simulink model "xy_platforma_fuzzy_test"  (Simulink 7.5)
settings: Solver=ode45  StartTime=0.0  StopTime=t_sim  RelTol=1e-3
values from neighbouring files (symbols this model uses):
  g = 9.81    [helikopter_maketa_paraametri.m]    (also in helikopter_maketa_parametri.m)
  Td = 0.1    [proo.m]
undefined symbols (not defined in the file or in its folder): a, ak_x, ak_y, Ax, Ay, const, d, Fc, freq_x, freq_y, Fs, Jl, K, K_komp, l, ml, period_x, period_y, phase_x, phase_y, phasedelay_x, phasedelay_y, pw_x, pw_y, R, r, t_step, vs, x0, x_poc_poz, x_step, y0, y_poc_poz, y_step
libraries: simulink x18, fuzblock x2
settings Model: Creator=Damjan  LastModifiedBy=Miha
settings DebuggingCC: SolverPrmCheckMsg=none

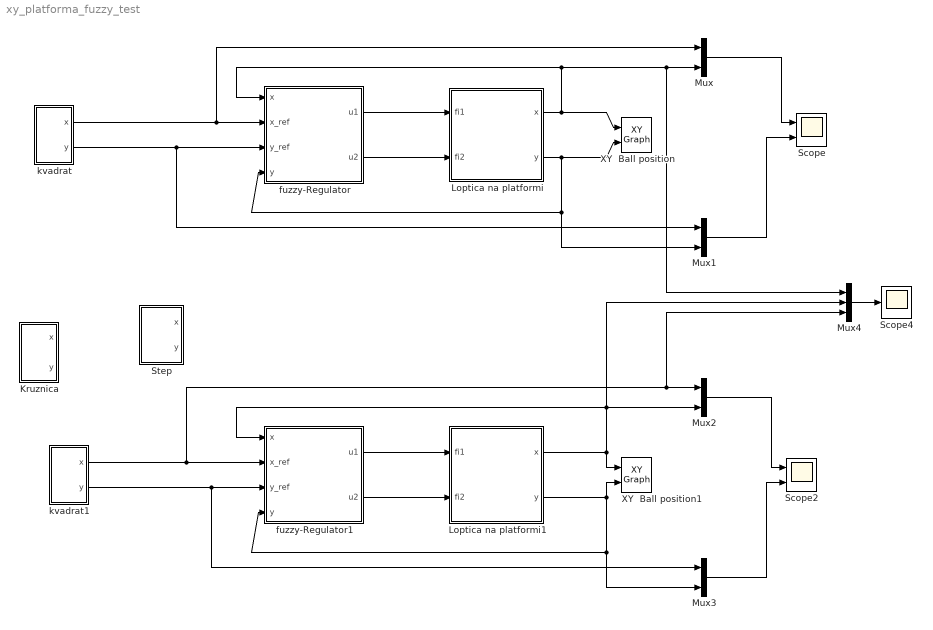
== system xy_platforma_fuzzy_test ==
  Kruznica : Subsystem
  Loptica na platformi : Subsystem
  Loptica na platformi1 : Subsystem
  Mux{,1..3} (4 alike) : Mux  Inputs=2
  Mux4 : Mux  Inputs=3
  Scope : Scope  NumInputPorts=2
      settings: YMin=0.15~0.15  YMax=0.2025~0.2025  SampleInput=on  SampleTime=1/25
  Scope2 : Scope  NumInputPorts=2
      settings: YMin=0.06~0.07  YMax=0.2~0.2  SaveName=ScopeData2  SampleInput=on  SampleTime=1/25
  Scope4 : Scope
      settings: TimeRange=4.054054054054055  YMin=0.115  YMax=0.22  SaveName=step  DataFormat=Array  MaxDataPoints=50000
  Step : Subsystem
  XY  Ball position : simulink/Sinks/XY Graph  SystemSampleTime=-1  xmin=0  xmax=0.3  ymin=0  ymax=0.3  st=-1
  XY  Ball position1 : simulink/Sinks/XY Graph  SystemSampleTime=-1  xmin=0  xmax=0.3  ymin=0  ymax=0.3  st=-1
  fuzzy-Regulator : Subsystem
  fuzzy-Regulator1 : Subsystem
  kvadrat : Subsystem
  kvadrat1 : Subsystem
  wires:
  Loptica na platformi/1(x) -> XY  Ball position/1, fuzzy-Regulator/1(x), Mux/2, Mux4/1
  Loptica na platformi/2(y) -> XY  Ball position/2, fuzzy-Regulator/4(y), Mux1/2
  Mux/1 -> Scope/1
  Mux1/1 -> Scope/2
  fuzzy-Regulator/1(u1) -> Loptica na platformi/1(fi1)
  fuzzy-Regulator/2(u2) -> Loptica na platformi/2(fi2)
  Loptica na platformi1/1(x) -> XY  Ball position1/1, fuzzy-Regulator1/1(x), Mux2/2, Mux4/2
  Loptica na platformi1/2(y) -> XY  Ball position1/2, fuzzy-Regulator1/4(y), Mux3/2
  Mux2/1 -> Scope2/1
  Mux3/1 -> Scope2/2
  fuzzy-Regulator1/1(u1) -> Loptica na platformi1/1(fi1)
  fuzzy-Regulator1/2(u2) -> Loptica na platformi1/2(fi2)
  kvadrat1/1(x) -> fuzzy-Regulator1/2(x_ref), Mux2/1, Mux4/3
  kvadrat1/2(y) -> fuzzy-Regulator1/3(y_ref), Mux3/1
  Mux4/1 -> Scope4/1
  kvadrat/1(x) -> fuzzy-Regulator/2(x_ref), Mux/1
  kvadrat/2(y) -> fuzzy-Regulator/3(y_ref), Mux1/1

== system xy_platforma_fuzzy_test/Kruznica ==
  sin x2 : Sin  Amplitude=Ax  Bias=x0  Frequency=freq_x  Phase=phase_x  Samples=10  SampleTime=0  Offset=0
  sin y2 : Sin  Amplitude=Ay  Bias=y0  Frequency=freq_y  Phase=phase_y  Samples=10  SampleTime=0  Offset=0
  x : Outport
  y : Outport  Port=2
  wires:
  sin x2/1 -> x/1
  sin y2/1 -> y/1

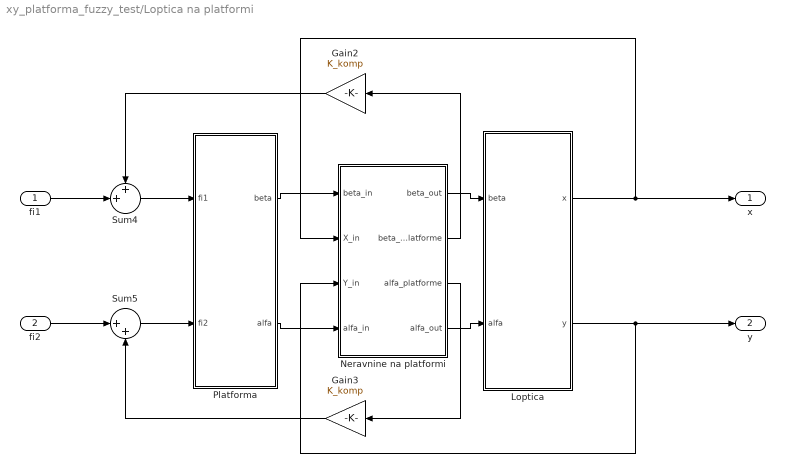
== system xy_platforma_fuzzy_test/Loptica na platformi ==
  fi1 : Inport
  fi2 : Inport  Port=2
  Gain2 : Gain  Gain=K_komp
  Gain3 : Gain  Gain=K_komp
  Loptica : Subsystem
  Neravnine na platformi : Subsystem
  Platforma : Subsystem
  Sum4 : Sum  Inputs=++|  RndMeth=Nearest
  Sum5 : Sum  Inputs=|++  RndMeth=Nearest
  x : Outport
  y : Outport  Port=2
  wires:
  Loptica/1(x) -> x/1, Neravnine na platformi/2(X_in)
  Platforma/1(beta) -> Neravnine na platformi/1(" beta_in")
  Platforma/2(alfa) -> Neravnine na platformi/4(alfa_in)
  Sum4/1 -> Platforma/1(fi1)
  Sum5/1 -> Platforma/2(fi2)
  Neravnine na platformi/3(alfa_platforme) -> Gain3/1
  Neravnine na platformi/2(beta_platforme) -> Gain2/1
  Loptica/2(y) -> y/1, Neravnine na platformi/3(Y_in)
  Neravnine na platformi/4(alfa_out) -> Loptica/2(alfa)
  Neravnine na platformi/1(beta_out) -> Loptica/1(beta)
  fi1/1 -> Sum4/2
  fi2/1 -> Sum5/1
  Gain2/1 -> Sum4/1
  Gain3/1 -> Sum5/2

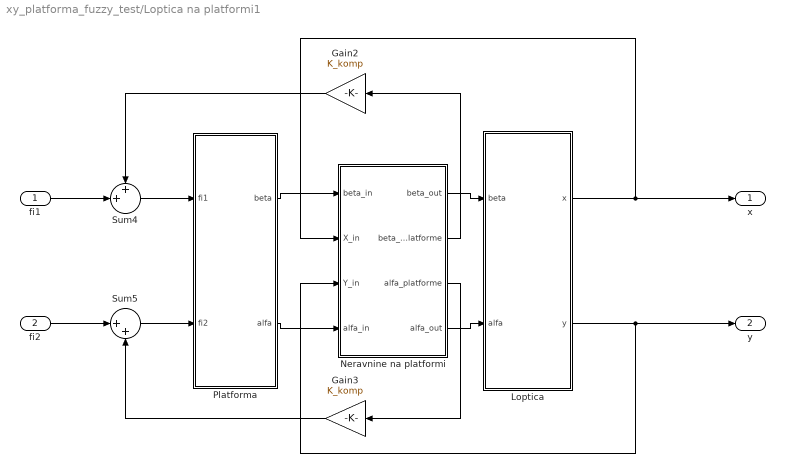
== system xy_platforma_fuzzy_test/Loptica na platformi1 ==
  fi1 : Inport
  fi2 : Inport  Port=2
  Gain2 : Gain  Gain=K_komp
  Gain3 : Gain  Gain=K_komp
  Loptica : Subsystem
  Neravnine na platformi : Subsystem
  Platforma : Subsystem
  Sum4 : Sum  Inputs=++|  RndMeth=Nearest
  Sum5 : Sum  Inputs=|++  RndMeth=Nearest
  x : Outport
  y : Outport  Port=2
  wires:
  Loptica/1(x) -> x/1, Neravnine na platformi/2(X_in)
  Platforma/1(beta) -> Neravnine na platformi/1(" beta_in")
  Platforma/2(alfa) -> Neravnine na platformi/4(alfa_in)
  Sum4/1 -> Platforma/1(fi1)
  Sum5/1 -> Platforma/2(fi2)
  Neravnine na platformi/3(alfa_platforme) -> Gain3/1
  Neravnine na platformi/2(beta_platforme) -> Gain2/1
  Loptica/2(y) -> y/1, Neravnine na platformi/3(Y_in)
  Neravnine na platformi/4(alfa_out) -> Loptica/2(alfa)
  Neravnine na platformi/1(beta_out) -> Loptica/1(beta)
  fi1/1 -> Sum4/2
  fi2/1 -> Sum5/1
  Gain2/1 -> Sum4/1
  Gain3/1 -> Sum5/2

== system xy_platforma_fuzzy_test/Step ==
  step1 : Step  Time=t_step  Before=x0  After=x_step  SampleTime=0
  step2 : Step  Time=t_step  Before=y0  After=y_step  SampleTime=0
  x : Outport
  y : Outport  Port=2
  wires:
  step1/1 -> x/1
  step2/1 -> y/1

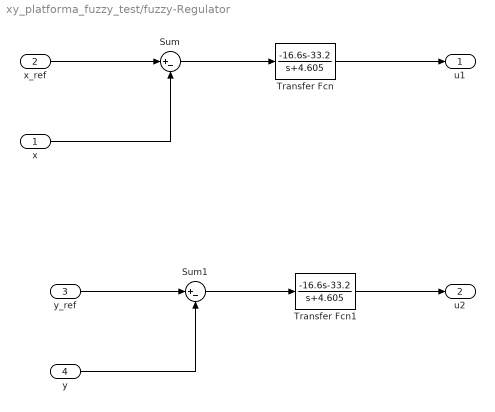
== system xy_platforma_fuzzy_test/fuzzy-Regulator ==
  x : Inport
  x_ref : Inport  Port=2
  y_ref : Inport  Port=3
  y : Inport  Port=4
  Sum : Sum  Inputs=|+-  OutDataType=fixdt(1, 16)  OutScaling=2^0
  Sum1 : Sum  Inputs=|+-  OutDataType=fixdt(1, 16)  OutScaling=2^0
  Transfer Fcn : TransferFcn  Numerator=[-16.6 -33.2]  Denominator=[1 4.605]
  Transfer Fcn1 : TransferFcn  Numerator=[-16.6 -33.2]  Denominator=[1 4.605]
  u1 : Outport
  u2 : Outport  Port=2
  wires:
  Transfer Fcn1/1 -> u2/1
  Transfer Fcn/1 -> u1/1
  x_ref/1 -> Sum/1
  x/1 -> Sum/2
  Sum/1 -> Transfer Fcn/1
  y_ref/1 -> Sum1/1
  y/1 -> Sum1/2
  Sum1/1 -> Transfer Fcn1/1

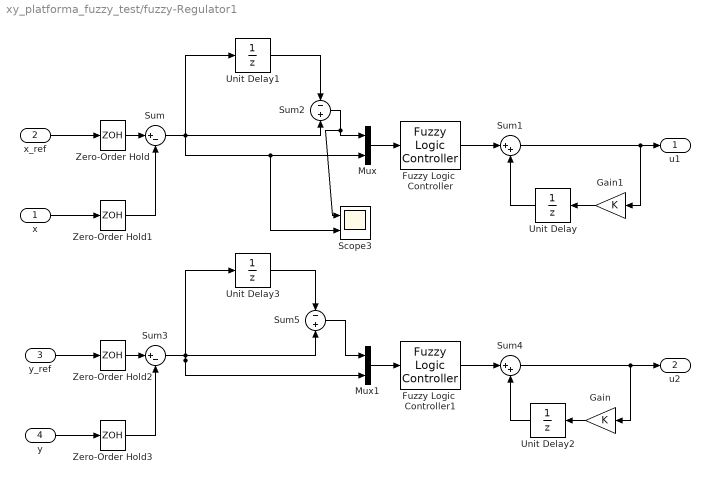
== system xy_platforma_fuzzy_test/fuzzy-Regulator1 ==
  x : Inport
  x_ref : Inport  Port=2
  y_ref : Inport  Port=3
  y : Inport  Port=4
  Fuzzy Logic  Controller : fuzblock/Fuzzy Logic  Controller  SystemSampleTime=-1  fis=fuzzyXY
  Fuzzy Logic  Controller1 : fuzblock/Fuzzy Logic  Controller  SystemSampleTime=-1  fis=fuzzyXY
  Gain : Gain  Gain=K  ParameterDataType=fixdt(1, 16)  ParameterScaling=2^0  OutDataType=fixdt(1, 16)  OutScaling=2^0
  Gain1 : Gain  Gain=K  ParameterDataType=fixdt(1, 16)  ParameterScaling=2^0  OutDataType=fixdt(1, 16)  OutScaling=2^0
  Mux : Mux  Inputs=2
  Mux1 : Mux  Inputs=2
  Scope3 : Scope  NumInputPorts=2
      settings: YMin=-0.015~-0.04  YMax=0.1~0.11  SaveName=ScopeData5  SampleInput=on  SampleTime=1/25
  Sum : Sum  Inputs=|+-
  Sum1 : Sum  Inputs=|++
  Sum2 : Sum  Inputs=-+
  Sum3 : Sum  Inputs=|+-
  Sum4 : Sum  Inputs=|++
  Sum5 : Sum  Inputs=-+
  Unit Delay{,1..3} (4 alike) : UnitDelay  SampleTime=Td
  Zero-Order Hold{,1..3} (4 alike) : ZeroOrderHold  SampleTime=Td
  u1 : Outport
  u2 : Outport  Port=2
  wires:
  Zero-Order Hold1/1 -> Sum/2
  Zero-Order Hold/1 -> Sum/1
  x_ref/1 -> Zero-Order Hold/1
  x/1 -> Zero-Order Hold1/1
  Fuzzy Logic  Controller/1 -> Sum1/1
  Unit Delay/1 -> Sum1/2
  Sum1/1 -> u1/1, Gain1/1
  Sum/1 -> Unit Delay1/1, Sum2/2, Mux/2, Scope3/2
  Mux/1 -> Fuzzy Logic  Controller/1
  Zero-Order Hold3/1 -> Sum3/2
  Zero-Order Hold2/1 -> Sum3/1
  y_ref/1 -> Zero-Order Hold2/1
  y/1 -> Zero-Order Hold3/1
  Fuzzy Logic  Controller1/1 -> Sum4/1
  Unit Delay2/1 -> Sum4/2
  Sum4/1 -> u2/1, Gain/1
  Sum3/1 -> Sum5/2, Mux1/2, Unit Delay3/1
  Mux1/1 -> Fuzzy Logic  Controller1/1
  Gain/1 -> Unit Delay2/1
  Gain1/1 -> Unit Delay/1
  Unit Delay1/1 -> Sum2/1
  Sum2/1 -> Mux/1, Scope3/1
  Unit Delay3/1 -> Sum5/1
  Sum5/1 -> Mux1/1

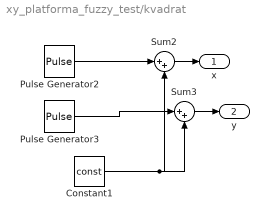
== system xy_platforma_fuzzy_test/kvadrat ==
  Constant1 : Constant  Value=const  OutDataType=fixdt(1, 16)  OutScaling=2^0
  Pulse Generator2 : DiscretePulseGenerator  PulseType=Time based  Amplitude=ak_x  Period=period_x  PulseWidth=pw_x  PhaseDelay=phasedelay_x  SampleTime=1
  Pulse Generator3 : DiscretePulseGenerator  PulseType=Time based  Amplitude=ak_y  Period=period_y  PulseWidth=pw_y  PhaseDelay=phasedelay_y  SampleTime=1
  Sum2 : Sum  Inputs=|++  OutDataType=fixdt(1, 16)  OutScaling=2^0
  Sum3 : Sum  Inputs=|++  OutDataType=fixdt(1, 16)  OutScaling=2^0
  x : Outport
  y : Outport  Port=2
  wires:
  Pulse Generator2/1 -> Sum2/1
  Pulse Generator3/1 -> Sum3/1
  Constant1/1 -> Sum3/2, Sum2/2
  Sum2/1 -> x/1
  Sum3/1 -> y/1

== system xy_platforma_fuzzy_test/kvadrat1 ==
  Constant1 : Constant  Value=const  OutDataType=fixdt(1, 16)  OutScaling=2^0
  Pulse Generator2 : DiscretePulseGenerator  PulseType=Time based  Amplitude=ak_x  Period=period_x  PulseWidth=pw_x  PhaseDelay=phasedelay_x  SampleTime=1
  Pulse Generator3 : DiscretePulseGenerator  PulseType=Time based  Amplitude=ak_y  Period=period_y  PulseWidth=pw_y  PhaseDelay=phasedelay_y  SampleTime=1
  Sum2 : Sum  Inputs=|++  OutDataType=fixdt(1, 16)  OutScaling=2^0
  Sum3 : Sum  Inputs=|++  OutDataType=fixdt(1, 16)  OutScaling=2^0
  x : Outport
  y : Outport  Port=2
  wires:
  Sum3/1 -> y/1
  Sum2/1 -> x/1
  Constant1/1 -> Sum2/2, Sum3/2
  Pulse Generator3/1 -> Sum3/1
  Pulse Generator2/1 -> Sum2/1

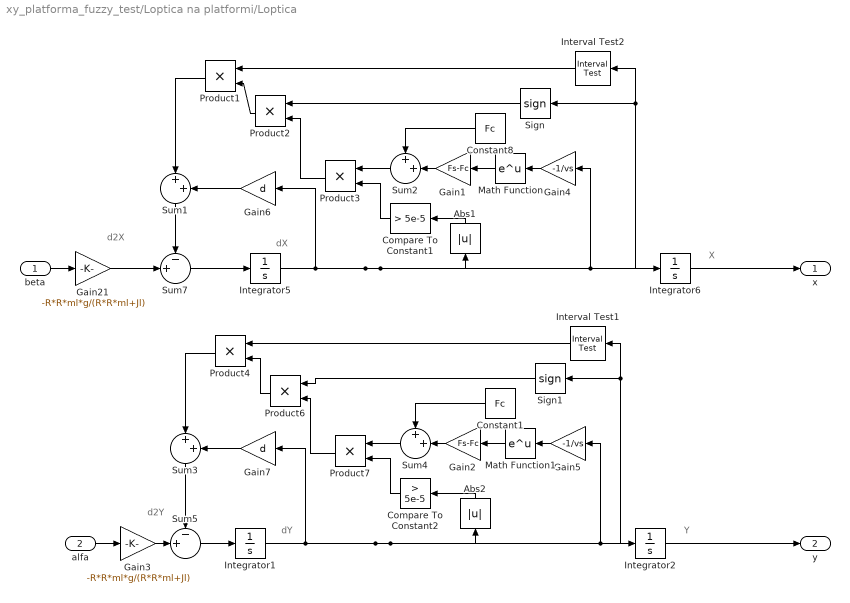
== system xy_platforma_fuzzy_test/Loptica na platformi/Loptica ==
  note: d2X
  note: dX
  note: X
  note: d2Y
  note: dY
  note: Y
  beta : Inport
  alfa : Inport  Port=2
  Abs1 : Abs
  Abs2 : Abs
  Compare To Constant1 : simulink/Logic and Bit Operations/Compare To Constant  SystemSampleTime=-1  relop=>  const=5e-5  LogicOutDataTypeMode=boolean  ZeroCross=off
  Compare To Constant2 : simulink/Logic and Bit Operations/Compare To Constant  SystemSampleTime=-1  relop=>  const=5e-5  LogicOutDataTypeMode=boolean  ZeroCross=off
  Constant1 : Constant  Value=Fc  SampleTime=0
  Constant8 : Constant  Value=Fc  SampleTime=0
  Gain1 : Gain  Gain=Fs-Fc  OutDataTypeStr=Inherit: Same as input  ParamDataTypeStr=Inherit: Same as input
  Gain2 : Gain  Gain=Fs-Fc  OutDataTypeStr=Inherit: Same as input  ParamDataTypeStr=Inherit: Same as input
  Gain21 : Gain  Gain=-R*R*ml*g/(R*R*ml+Jl)
  Gain3 : Gain  Gain=-R*R*ml*g/(R*R*ml+Jl)
  Gain4 : Gain  Gain=-1/vs  OutDataTypeStr=Inherit: Same as input  ParamDataTypeStr=Inherit: Same as input
  Gain5 : Gain  Gain=-1/vs  OutDataTypeStr=Inherit: Same as input  ParamDataTypeStr=Inherit: Same as input
  Gain6 : Gain  Gain=d  OutDataTypeStr=Inherit: Same as input  ParamDataTypeStr=Inherit: Same as input
  Gain7 : Gain  Gain=d  OutDataTypeStr=Inherit: Same as input  ParamDataTypeStr=Inherit: Same as input
  Integrator1 : Integrator
  Integrator2 : Integrator  InitialCondition=y_poc_poz
  Integrator5 : Integrator
  Integrator6 : Integrator  InitialCondition=x_poc_poz
  Interval Test1 : simulink/Logic and Bit Operations/Interval Test  SystemSampleTime=-1  IntervalClosedRight=on  uplimit=5e-5  IntervalClosedLeft=on  lowlimit=-5e-5  LogicOutDataTypeMode=boolean
  Interval Test2 : simulink/Logic and Bit Operations/Interval Test  SystemSampleTime=-1  IntervalClosedRight=on  uplimit=5e-5  IntervalClosedLeft=on  lowlimit=-5e-5  LogicOutDataTypeMode=boolean
  Math Function : Math  SaturateOnIntegerOverflow=on
  Math Function1 : Math  SaturateOnIntegerOverflow=on
  Product{1..4,6..7} (6 alike) : Product  RndMeth=Zero
  Sign : Signum
  Sign1 : Signum
  Sum1 : Sum  Inputs=|++
  Sum2 : Sum  Inputs=++|
  Sum3 : Sum  Inputs=|++
  Sum4 : Sum  Inputs=++|
  Sum5 : Sum  Inputs=-+|
  Sum7 : Sum  Inputs=-+|
  x : Outport
  y : Outport  Port=2
  wires:
  beta/1 -> Gain21/1
  Integrator5/1 -> Gain6/1, Abs1/1, Integrator6/1, Interval Test2/1, Sign/1, Gain4/1
  Sum7/1 -> Integrator5/1
  Gain4/1 -> Math Function/1
  Math Function/1 -> Gain1/1
  Gain1/1 -> Sum2/2
  Constant8/1 -> Sum2/1
  Sign/1 -> Product2/1
  Abs1/1 -> Compare To Constant1/1
  Sum2/1 -> Product3/1
  Compare To Constant1/1 -> Product3/2
  Product3/1 -> Product2/2
  Integrator1/1 -> Gain5/1, Sign1/1, Interval Test1/1, Integrator2/1, Abs2/1, Gain7/1
  Gain3/1 -> Sum5/2
  Sum5/1 -> Integrator1/1
  Gain5/1 -> Math Function1/1
  Math Function1/1 -> Gain2/1
  Gain2/1 -> Sum4/2
  Constant1/1 -> Sum4/1
  Sign1/1 -> Product6/1
  Abs2/1 -> Compare To Constant2/1
  Sum4/1 -> Product7/1
  Compare To Constant2/1 -> Product7/2
  Product7/1 -> Product6/2
  alfa/1 -> Gain3/1
  Integrator6/1 -> x/1
  Integrator2/1 -> y/1
  Interval Test2/1 -> Product1/1
  Product2/1 -> Product1/2
  Gain21/1 -> Sum7/2
  Product6/1 -> Product4/2
  Interval Test1/1 -> Product4/1
  Gain6/1 -> Sum1/2
  Sum1/1 -> Sum7/1
  Gain7/1 -> Sum3/2
  Sum3/1 -> Sum5/1
  Product1/1 -> Sum1/1
  Product4/1 -> Sum3/1

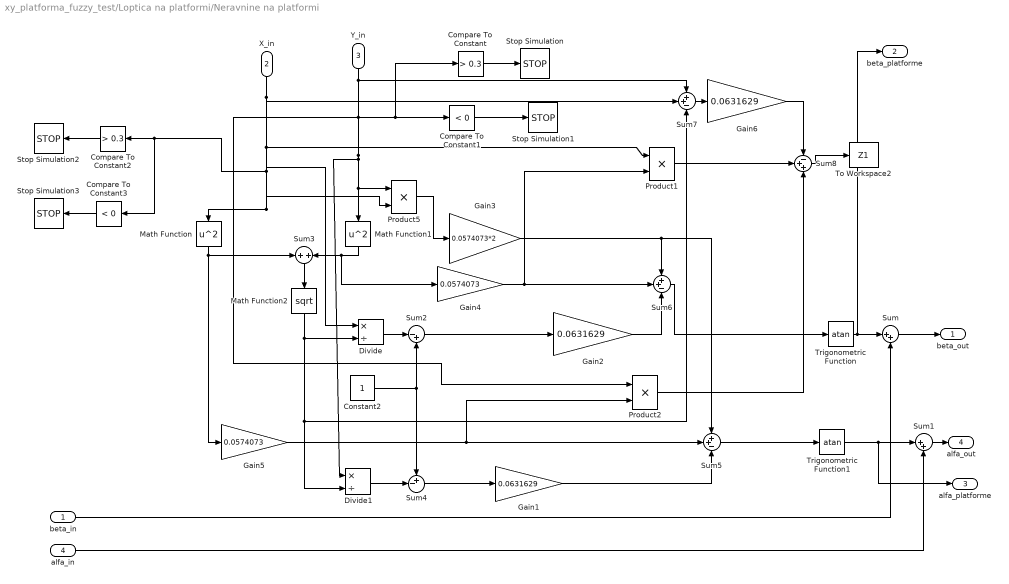
== system xy_platforma_fuzzy_test/Loptica na platformi/Neravnine na platformi ==
  " beta_in" : Inport
  X_in : Inport  Port=2
  Y_in : Inport  Port=3
  alfa_in : Inport  Port=4
  Compare To Constant : simulink/Logic and Bit Operations/Compare To Constant  SystemSampleTime=-1  relop=>  const=0.3  LogicOutDataTypeMode=boolean  ZeroCross=off
  Compare To Constant1 : simulink/Logic and Bit Operations/Compare To Constant  SystemSampleTime=-1  relop=<  const=0  LogicOutDataTypeMode=boolean  ZeroCross=off
  Compare To Constant2 : simulink/Logic and Bit Operations/Compare To Constant  SystemSampleTime=-1  relop=>  const=0.3  LogicOutDataTypeMode=boolean  ZeroCross=off
  Compare To Constant3 : simulink/Logic and Bit Operations/Compare To Constant  SystemSampleTime=-1  relop=<  const=0  LogicOutDataTypeMode=boolean  ZeroCross=off
  Constant2 : Constant  SampleTime=0
  Divide : Product  Inputs=*/
  Divide1 : Product  Inputs=*/
  Gain1 : Gain  Gain=0.0631629
  Gain2 : Gain  Gain=0.0631629
  Gain3 : Gain  Gain=0.0574073*2
  Gain4 : Gain  Gain=0.0574073
  Gain5 : Gain  Gain=0.0574073
  Gain6 : Gain  Gain=0.0631629
  Math Function : Math  Operator=square  SaturateOnIntegerOverflow=on
  Math Function1 : Math  Operator=square  SaturateOnIntegerOverflow=on
  Math Function2 : Math  Operator=sqrt  SaturateOnIntegerOverflow=on
  Product1 : Product  RndMeth=Zero
  Product2 : Product  RndMeth=Zero
  Product5 : Product  RndMeth=Zero
  Stop Simulation{,1..3} (4 alike) : Stop
  Sum : Sum  Inputs=|++
  Sum1 : Sum  Inputs=|++
  Sum2 : Sum  Inputs=|-+
  Sum3 : Sum
  Sum4 : Sum  Inputs=+-|
  Sum5 : Sum  Inputs=++-
  Sum6 : Sum  Inputs=++-
  Sum7 : Sum  Inputs=++-
  Sum8 : Sum  Inputs=-++
  To Workspace2 : ToWorkspace  VariableName=Z1  SampleTime=-1  SaveFormat=Array
  Trigonometric Function : Trigonometry  Operator=atan
  Trigonometric Function1 : Trigonometry  Operator=atan
  beta_out : Outport
  beta_platforme : Outport  Port=2
  alfa_platforme : Outport  Port=3
  alfa_out : Outport  Port=4
  wires:
  Sum/1 -> beta_out/1
  Sum1/1 -> alfa_out/1
  " beta_in"/1 -> Sum/2
  alfa_in/1 -> Sum1/2
  Trigonometric Function/1 -> beta_platforme/1, Sum/1
  Trigonometric Function1/1 -> Sum1/1, alfa_platforme/1
  X_in/1 -> Compare To Constant2/1, Compare To Constant3/1, Divide/1, Math Function/1, Product5/2, Product1/1, Sum7/2
  Y_in/1 -> Compare To Constant/1, Compare To Constant1/1, Divide1/1, Math Function1/1, Product5/1, Product2/1, Sum7/1
  Math Function/1 -> Sum3/1, Gain5/1
  Math Function1/1 -> Sum3/2, Gain4/1
  Sum3/1 -> Math Function2/1
  Math Function2/1 -> Divide/2, Divide1/2, Sum7/3
  Divide/1 -> Sum2/1
  Constant2/1 -> Sum2/2, Sum4/1
  Sum2/1 -> Gain2/1
  Divide1/1 -> Sum4/2
  Sum4/1 -> Gain1/1
  Product5/1 -> Gain3/1
  Gain4/1 -> Sum6/2, Product1/2
  Gain3/1 -> Sum6/1, Sum5/1
  Sum6/1 -> Trigonometric Function/1
  Gain1/1 -> Sum5/3
  Gain5/1 -> Sum5/2, Product2/2
  Sum5/1 -> Trigonometric Function1/1
  Sum7/1 -> Gain6/1
  Product1/1 -> Sum8/2
  Product2/1 -> Sum8/3
  Sum8/1 -> To Workspace2/1
  Gain6/1 -> Sum8/1
  Compare To Constant2/1 -> Stop Simulation2/1
  Compare To Constant3/1 -> Stop Simulation3/1
  Compare To Constant/1 -> Stop Simulation/1
  Compare To Constant1/1 -> Stop Simulation1/1
  Gain2/1 -> Sum6/3

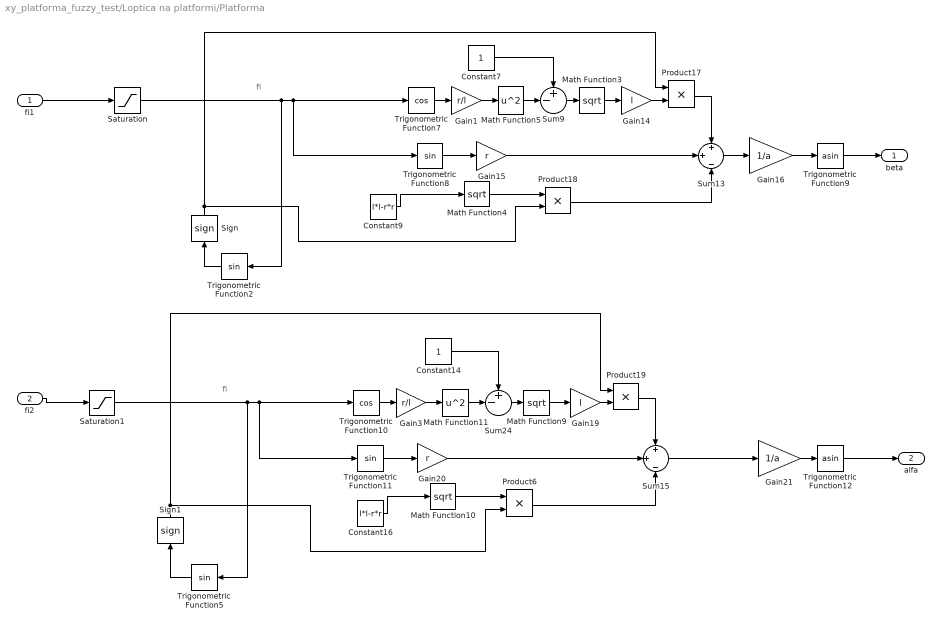
== system xy_platforma_fuzzy_test/Loptica na platformi/Platforma ==
  note: fi
  note: fi
  fi1 : Inport
  fi2 : Inport  Port=2
  Constant14 : Constant  SampleTime=0
  Constant16 : Constant  Value=l*l-r*r  SampleTime=0
  Constant7 : Constant  SampleTime=0
  Constant9 : Constant  Value=l*l-r*r  SampleTime=0
  Gain1 : Gain  Gain=r/l
  Gain14 : Gain  Gain=l
  Gain15 : Gain  Gain=r
  Gain16 : Gain  Gain=1/a
  Gain19 : Gain  Gain=l
  Gain20 : Gain  Gain=r
  Gain21 : Gain  Gain=1/a
  Gain3 : Gain  Gain=r/l
  Math Function{3..4,9..10} (4 alike) : Math  Operator=sqrt  SaturateOnIntegerOverflow=on
  Math Function11 : Math  Operator=square  SaturateOnIntegerOverflow=on
  Math Function5 : Math  Operator=square  SaturateOnIntegerOverflow=on
  Product{6,17..19} (4 alike) : Product  RndMeth=Zero
  Saturation : Saturate  UpperLimit=pi/2  LowerLimit=-pi/2
  Saturation1 : Saturate  UpperLimit=pi/2  LowerLimit=-pi/2
  Sign : Signum  ZeroCross=off
  Sign1 : Signum  ZeroCross=off
  Sum13 : Sum  Inputs=+|+|-  InputSameDT=on
  Sum15 : Sum  Inputs=+|+|-  InputSameDT=on
  Sum24 : Sum  Inputs=+-|
  Sum9 : Sum  Inputs=+-|
  Trigonometric Function10 : Trigonometry  Operator=cos
  Trigonometric Function{2,5,8,11} (4 alike) : Trigonometry
  Trigonometric Function12 : Trigonometry  Operator=asin
  Trigonometric Function7 : Trigonometry  Operator=cos
  Trigonometric Function9 : Trigonometry  Operator=asin
  beta : Outport
  alfa : Outport  Port=2
  wires:
  fi1/1 -> Saturation/1
  Trigonometric Function2/1 -> Sign/1
  Sign/1 -> Product18/2, Product17/1
  Trigonometric Function7/1 -> Gain1/1
  Constant7/1 -> Sum9/1
  Gain1/1 -> Math Function5/1
  Sum9/1 -> Math Function3/1
  Math Function3/1 -> Gain14/1
  Trigonometric Function8/1 -> Gain15/1
  Gain15/1 -> Sum13/2
  Constant9/1 -> Math Function4/1
  Gain16/1 -> Trigonometric Function9/1
  Math Function5/1 -> Sum9/2
  Sum13/1 -> Gain16/1
  Trigonometric Function5/1 -> Sign1/1
  Sign1/1 -> Product6/2, Product19/1
  Trigonometric Function10/1 -> Gain3/1
  Constant14/1 -> Sum24/1
  Gain3/1 -> Math Function11/1
  Sum24/1 -> Math Function9/1
  Math Function9/1 -> Gain19/1
  Trigonometric Function11/1 -> Gain20/1
  Gain20/1 -> Sum15/2
  Constant16/1 -> Math Function10/1
  Math Function11/1 -> Sum24/2
  Gain21/1 -> Trigonometric Function12/1
  Product17/1 -> Sum13/1
  Gain14/1 -> Product17/2
  Product18/1 -> Sum13/3
  Math Function4/1 -> Product18/1
  Product19/1 -> Sum15/1
  Gain19/1 -> Product19/2
  Product6/1 -> Sum15/3
  Math Function10/1 -> Product6/1
  Sum15/1 -> Gain21/1
  fi2/1 -> Saturation1/1
  Trigonometric Function9/1 -> beta/1
  Trigonometric Function12/1 -> alfa/1
  Saturation/1 -> Trigonometric Function7/1, Trigonometric Function8/1, Trigonometric Function2/1
  Saturation1/1 -> Trigonometric Function11/1, Trigonometric Function10/1, Trigonometric Function5/1

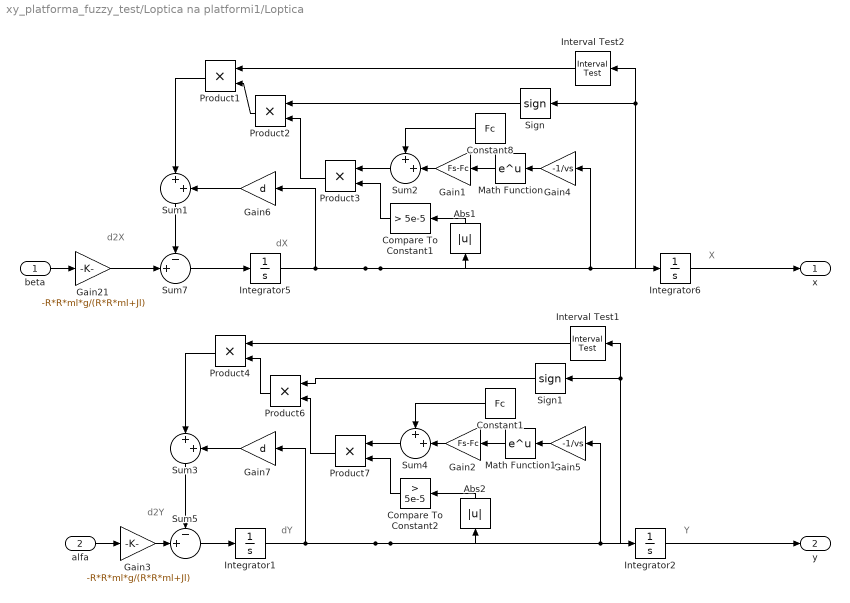
== system xy_platforma_fuzzy_test/Loptica na platformi1/Loptica ==
  note: d2X
  note: dX
  note: X
  note: d2Y
  note: dY
  note: Y
  beta : Inport
  alfa : Inport  Port=2
  Abs1 : Abs
  Abs2 : Abs
  Compare To Constant1 : simulink/Logic and Bit Operations/Compare To Constant  SystemSampleTime=-1  relop=>  const=5e-5  LogicOutDataTypeMode=boolean  ZeroCross=off
  Compare To Constant2 : simulink/Logic and Bit Operations/Compare To Constant  SystemSampleTime=-1  relop=>  const=5e-5  LogicOutDataTypeMode=boolean  ZeroCross=off
  Constant1 : Constant  Value=Fc  SampleTime=0
  Constant8 : Constant  Value=Fc  SampleTime=0
  Gain1 : Gain  Gain=Fs-Fc  OutDataTypeStr=Inherit: Same as input  ParamDataTypeStr=Inherit: Same as input
  Gain2 : Gain  Gain=Fs-Fc  OutDataTypeStr=Inherit: Same as input  ParamDataTypeStr=Inherit: Same as input
  Gain21 : Gain  Gain=-R*R*ml*g/(R*R*ml+Jl)
  Gain3 : Gain  Gain=-R*R*ml*g/(R*R*ml+Jl)
  Gain4 : Gain  Gain=-1/vs  OutDataTypeStr=Inherit: Same as input  ParamDataTypeStr=Inherit: Same as input
  Gain5 : Gain  Gain=-1/vs  OutDataTypeStr=Inherit: Same as input  ParamDataTypeStr=Inherit: Same as input
  Gain6 : Gain  Gain=d  OutDataTypeStr=Inherit: Same as input  ParamDataTypeStr=Inherit: Same as input
  Gain7 : Gain  Gain=d  OutDataTypeStr=Inherit: Same as input  ParamDataTypeStr=Inherit: Same as input
  Integrator1 : Integrator
  Integrator2 : Integrator  InitialCondition=y_poc_poz
  Integrator5 : Integrator
  Integrator6 : Integrator  InitialCondition=x_poc_poz
  Interval Test1 : simulink/Logic and Bit Operations/Interval Test  SystemSampleTime=-1  IntervalClosedRight=on  uplimit=5e-5  IntervalClosedLeft=on  lowlimit=-5e-5  LogicOutDataTypeMode=boolean
  Interval Test2 : simulink/Logic and Bit Operations/Interval Test  SystemSampleTime=-1  IntervalClosedRight=on  uplimit=5e-5  IntervalClosedLeft=on  lowlimit=-5e-5  LogicOutDataTypeMode=boolean
  Math Function : Math  SaturateOnIntegerOverflow=on
  Math Function1 : Math  SaturateOnIntegerOverflow=on
  Product{1..4,6..7} (6 alike) : Product  RndMeth=Zero
  Sign : Signum
  Sign1 : Signum
  Sum1 : Sum  Inputs=|++
  Sum2 : Sum  Inputs=++|
  Sum3 : Sum  Inputs=|++
  Sum4 : Sum  Inputs=++|
  Sum5 : Sum  Inputs=-+|
  Sum7 : Sum  Inputs=-+|
  x : Outport
  y : Outport  Port=2
  wires:
  beta/1 -> Gain21/1
  Integrator5/1 -> Gain6/1, Abs1/1, Integrator6/1, Interval Test2/1, Sign/1, Gain4/1
  Sum7/1 -> Integrator5/1
  Gain4/1 -> Math Function/1
  Math Function/1 -> Gain1/1
  Gain1/1 -> Sum2/2
  Constant8/1 -> Sum2/1
  Sign/1 -> Product2/1
  Abs1/1 -> Compare To Constant1/1
  Sum2/1 -> Product3/1
  Compare To Constant1/1 -> Product3/2
  Product3/1 -> Product2/2
  Integrator1/1 -> Gain5/1, Sign1/1, Interval Test1/1, Integrator2/1, Abs2/1, Gain7/1
  Gain3/1 -> Sum5/2
  Sum5/1 -> Integrator1/1
  Gain5/1 -> Math Function1/1
  Math Function1/1 -> Gain2/1
  Gain2/1 -> Sum4/2
  Constant1/1 -> Sum4/1
  Sign1/1 -> Product6/1
  Abs2/1 -> Compare To Constant2/1
  Sum4/1 -> Product7/1
  Compare To Constant2/1 -> Product7/2
  Product7/1 -> Product6/2
  alfa/1 -> Gain3/1
  Integrator6/1 -> x/1
  Integrator2/1 -> y/1
  Interval Test2/1 -> Product1/1
  Product2/1 -> Product1/2
  Gain21/1 -> Sum7/2
  Product6/1 -> Product4/2
  Interval Test1/1 -> Product4/1
  Gain6/1 -> Sum1/2
  Sum1/1 -> Sum7/1
  Gain7/1 -> Sum3/2
  Sum3/1 -> Sum5/1
  Product1/1 -> Sum1/1
  Product4/1 -> Sum3/1

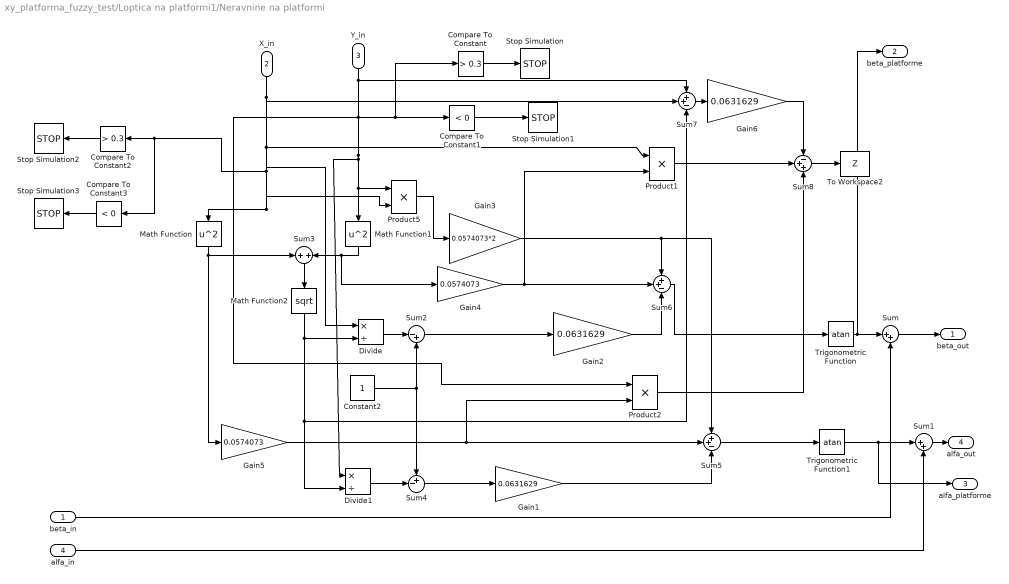
== system xy_platforma_fuzzy_test/Loptica na platformi1/Neravnine na platformi ==
  " beta_in" : Inport
  X_in : Inport  Port=2
  Y_in : Inport  Port=3
  alfa_in : Inport  Port=4
  Compare To Constant : simulink/Logic and Bit Operations/Compare To Constant  SystemSampleTime=-1  relop=>  const=0.3  LogicOutDataTypeMode=boolean  ZeroCross=off
  Compare To Constant1 : simulink/Logic and Bit Operations/Compare To Constant  SystemSampleTime=-1  relop=<  const=0  LogicOutDataTypeMode=boolean  ZeroCross=off
  Compare To Constant2 : simulink/Logic and Bit Operations/Compare To Constant  SystemSampleTime=-1  relop=>  const=0.3  LogicOutDataTypeMode=boolean  ZeroCross=off
  Compare To Constant3 : simulink/Logic and Bit Operations/Compare To Constant  SystemSampleTime=-1  relop=<  const=0  LogicOutDataTypeMode=boolean  ZeroCross=off
  Constant2 : Constant  SampleTime=0
  Divide : Product  Inputs=*/
  Divide1 : Product  Inputs=*/
  Gain1 : Gain  Gain=0.0631629
  Gain2 : Gain  Gain=0.0631629
  Gain3 : Gain  Gain=0.0574073*2
  Gain4 : Gain  Gain=0.0574073
  Gain5 : Gain  Gain=0.0574073
  Gain6 : Gain  Gain=0.0631629
  Math Function : Math  Operator=square  SaturateOnIntegerOverflow=on
  Math Function1 : Math  Operator=square  SaturateOnIntegerOverflow=on
  Math Function2 : Math  Operator=sqrt  SaturateOnIntegerOverflow=on
  Product1 : Product  RndMeth=Zero
  Product2 : Product  RndMeth=Zero
  Product5 : Product  RndMeth=Zero
  Stop Simulation{,1..3} (4 alike) : Stop
  Sum : Sum  Inputs=|++
  Sum1 : Sum  Inputs=|++
  Sum2 : Sum  Inputs=|-+
  Sum3 : Sum
  Sum4 : Sum  Inputs=+-|
  Sum5 : Sum  Inputs=++-
  Sum6 : Sum  Inputs=++-
  Sum7 : Sum  Inputs=++-
  Sum8 : Sum  Inputs=-++
  To Workspace2 : ToWorkspace  VariableName=Z  SampleTime=-1  SaveFormat=Array
  Trigonometric Function : Trigonometry  Operator=atan
  Trigonometric Function1 : Trigonometry  Operator=atan
  beta_out : Outport
  beta_platforme : Outport  Port=2
  alfa_platforme : Outport  Port=3
  alfa_out : Outport  Port=4
  wires:
  Sum/1 -> beta_out/1
  Sum1/1 -> alfa_out/1
  " beta_in"/1 -> Sum/2
  alfa_in/1 -> Sum1/2
  Trigonometric Function/1 -> beta_platforme/1, Sum/1
  Trigonometric Function1/1 -> Sum1/1, alfa_platforme/1
  X_in/1 -> Compare To Constant2/1, Compare To Constant3/1, Divide/1, Math Function/1, Product5/2, Product1/1, Sum7/2
  Y_in/1 -> Compare To Constant/1, Compare To Constant1/1, Divide1/1, Math Function1/1, Product5/1, Product2/1, Sum7/1
  Math Function/1 -> Sum3/1, Gain5/1
  Math Function1/1 -> Sum3/2, Gain4/1
  Sum3/1 -> Math Function2/1
  Math Function2/1 -> Divide/2, Divide1/2, Sum7/3
  Divide/1 -> Sum2/1
  Constant2/1 -> Sum2/2, Sum4/1
  Sum2/1 -> Gain2/1
  Divide1/1 -> Sum4/2
  Sum4/1 -> Gain1/1
  Product5/1 -> Gain3/1
  Gain4/1 -> Sum6/2, Product1/2
  Gain3/1 -> Sum6/1, Sum5/1
  Sum6/1 -> Trigonometric Function/1
  Gain1/1 -> Sum5/3
  Gain5/1 -> Sum5/2, Product2/2
  Sum5/1 -> Trigonometric Function1/1
  Sum7/1 -> Gain6/1
  Product1/1 -> Sum8/2
  Product2/1 -> Sum8/3
  Sum8/1 -> To Workspace2/1
  Gain6/1 -> Sum8/1
  Compare To Constant2/1 -> Stop Simulation2/1
  Compare To Constant3/1 -> Stop Simulation3/1
  Compare To Constant/1 -> Stop Simulation/1
  Compare To Constant1/1 -> Stop Simulation1/1
  Gain2/1 -> Sum6/3

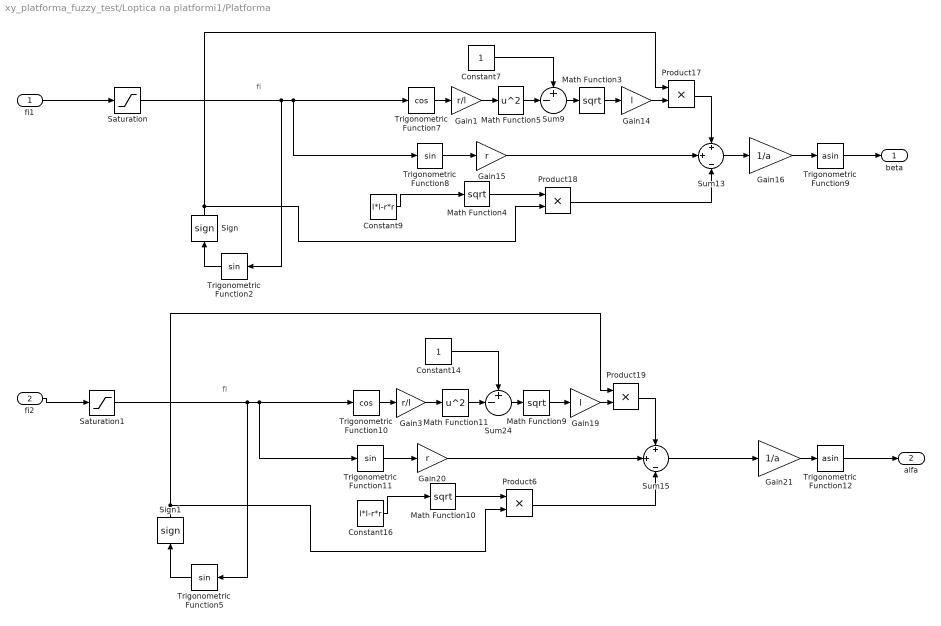
== system xy_platforma_fuzzy_test/Loptica na platformi1/Platforma ==
  note: fi
  note: fi
  fi1 : Inport
  fi2 : Inport  Port=2
  Constant14 : Constant  SampleTime=0
  Constant16 : Constant  Value=l*l-r*r  SampleTime=0
  Constant7 : Constant  SampleTime=0
  Constant9 : Constant  Value=l*l-r*r  SampleTime=0
  Gain1 : Gain  Gain=r/l
  Gain14 : Gain  Gain=l
  Gain15 : Gain  Gain=r
  Gain16 : Gain  Gain=1/a
  Gain19 : Gain  Gain=l
  Gain20 : Gain  Gain=r
  Gain21 : Gain  Gain=1/a
  Gain3 : Gain  Gain=r/l
  Math Function{3..4,9..10} (4 alike) : Math  Operator=sqrt  SaturateOnIntegerOverflow=on
  Math Function11 : Math  Operator=square  SaturateOnIntegerOverflow=on
  Math Function5 : Math  Operator=square  SaturateOnIntegerOverflow=on
  Product{6,17..19} (4 alike) : Product  RndMeth=Zero
  Saturation : Saturate  UpperLimit=pi/2  LowerLimit=-pi/2
  Saturation1 : Saturate  UpperLimit=pi/2  LowerLimit=-pi/2
  Sign : Signum  ZeroCross=off
  Sign1 : Signum  ZeroCross=off
  Sum13 : Sum  Inputs=+|+|-  InputSameDT=on
  Sum15 : Sum  Inputs=+|+|-  InputSameDT=on
  Sum24 : Sum  Inputs=+-|
  Sum9 : Sum  Inputs=+-|
  Trigonometric Function10 : Trigonometry  Operator=cos
  Trigonometric Function{2,5,8,11} (4 alike) : Trigonometry
  Trigonometric Function12 : Trigonometry  Operator=asin
  Trigonometric Function7 : Trigonometry  Operator=cos
  Trigonometric Function9 : Trigonometry  Operator=asin
  beta : Outport
  alfa : Outport  Port=2
  wires:
  fi1/1 -> Saturation/1
  Trigonometric Function2/1 -> Sign/1
  Sign/1 -> Product18/2, Product17/1
  Trigonometric Function7/1 -> Gain1/1
  Constant7/1 -> Sum9/1
  Gain1/1 -> Math Function5/1
  Sum9/1 -> Math Function3/1
  Math Function3/1 -> Gain14/1
  Trigonometric Function8/1 -> Gain15/1
  Gain15/1 -> Sum13/2
  Constant9/1 -> Math Function4/1
  Gain16/1 -> Trigonometric Function9/1
  Math Function5/1 -> Sum9/2
  Sum13/1 -> Gain16/1
  Trigonometric Function5/1 -> Sign1/1
  Sign1/1 -> Product6/2, Product19/1
  Trigonometric Function10/1 -> Gain3/1
  Constant14/1 -> Sum24/1
  Gain3/1 -> Math Function11/1
  Sum24/1 -> Math Function9/1
  Math Function9/1 -> Gain19/1
  Trigonometric Function11/1 -> Gain20/1
  Gain20/1 -> Sum15/2
  Constant16/1 -> Math Function10/1
  Math Function11/1 -> Sum24/2
  Gain21/1 -> Trigonometric Function12/1
  Product17/1 -> Sum13/1
  Gain14/1 -> Product17/2
  Product18/1 -> Sum13/3
  Math Function4/1 -> Product18/1
  Product19/1 -> Sum15/1
  Gain19/1 -> Product19/2
  Product6/1 -> Sum15/3
  Math Function10/1 -> Product6/1
  Sum15/1 -> Gain21/1
  fi2/1 -> Saturation1/1
  Trigonometric Function9/1 -> beta/1
  Trigonometric Function12/1 -> alfa/1
  Saturation/1 -> Trigonometric Function7/1, Trigonometric Function8/1, Trigonometric Function2/1
  Saturation1/1 -> Trigonometric Function11/1, Trigonometric Function10/1, Trigonometric Function5/1
